simulink model "Punto_6b"  (R2022a)
settings: Solver=VariableStepAuto  StartTime=0.0  StopTime=10.0  RelTol=1e-3
undefined symbols (not defined in the file): A, B
settings Model: Creator=garzo  LastModifiedBy=garzo

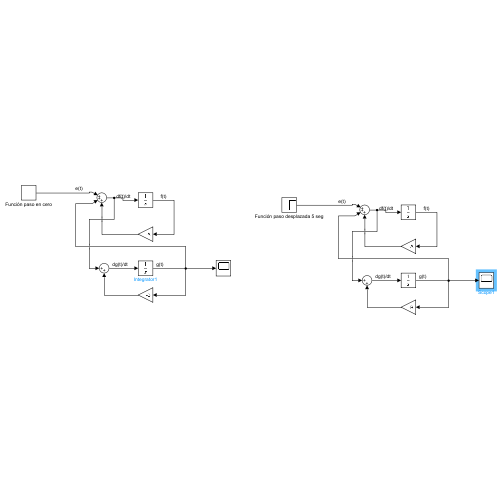
[thumbnail: Simulink's stored preview of the top-level diagram]
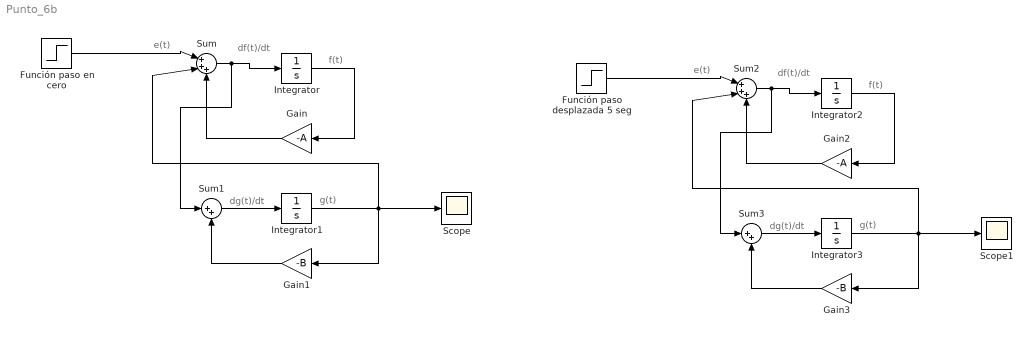
== system Punto_6b ==
  note: g(t)
  note: e(t)
  note: f(t)
  note: dg(t)/dt
  note: df(t)/dt
  note: g(t)
  note: f(t)
  note: df(t)/dt
  note: e(t)
  note: dg(t)/dt
  Función paso desplazada 5 seg : Step  Time=5  SampleTime=0
  Función paso en cero : Step  Time=0  SampleTime=0
  Gain : Gain  Gain=-A
  Gain1 : Gain  Gain=-B
  Gain2 : Gain  Gain=-A
  Gain3 : Gain  Gain=-B
  Integrator{,1..3} (4 alike) : Integrator
  Scope : Scope
  Scope1 : Scope
  Sum : Sum  Inputs=|+++
  Sum1 : Sum  Inputs=|++
  Sum2 : Sum  Inputs=|+++
  Sum3 : Sum  Inputs=|++
  wires:
  Integrator1/1 -> Scope/1, Sum/2, Gain1/1
  Sum1/1 -> Integrator1/1
  Gain1/1 -> Sum1/2
  Integrator/1 -> Gain/1
  Gain/1 -> Sum/3
  Sum/1 -> Sum1/1, Integrator/1
  Función paso en cero/1 -> Sum/1
  Sum2/1 -> Sum3/1, Integrator2/1
  Gain3/1 -> Sum3/2
  Integrator3/1 -> Scope1/1, Sum2/2, Gain3/1
  Integrator2/1 -> Gain2/1
  Sum3/1 -> Integrator3/1
  Gain2/1 -> Sum2/3
  Función paso desplazada 5 seg/1 -> Sum2/1
